simulink model "Sender"  (R2023a)
settings: Solver=FixedStepAuto  StartTime=0.0  StopTime=inf  RelTol=1e-3
undefined symbols (not defined in the file): DISTANCE, FINAL_1
libraries: androidaudiovideolib x4, simulink_extras x4, androidcommunicationlib x4, androiduilib x2, dspswit3 x2, androidsensorlib x2
settings Model: Creator=mohit  LastModifiedBy=mohit
settings OptimizationCC: EnhancedBackFolding=on  PassReuseOutputArgsAs=Individual arguments  ZeroExternalMemoryAtStartup=off  ZeroInternalMemoryAtStartup=off  MaxStackSize=64  OptimizeBlockOrder=speed  DifferentSizesBufferReuse=on  OptimizationCustomize=off  EfficientTunableParamExpr=on
settings DebuggingCC: ParameterTunabilityLossMsg=error
settings HardwareCC: ProdBitPerPointer=32  ProdBitPerSizeT=32  ProdBitPerPtrDiffT=32  ProdLargestAtomicInteger=Long  ProdLargestAtomicFloat=Double  ProdWordSize=32  ProdHWDeviceType=ARM Compatible->ARM Cortex  UseEmbeddedCoderFeatures=off  UseSimulinkCoderFeatures=off
settings SFSimCC: MATLABDynamicMemAlloc=off
settings RTWCC: Description=Embedded Coder  SystemTargetFile=ert.tlc  HardwareBoard=Android Device  TLCOptions="-aInlineSetEventsForThisBaseRateFcn=TLC_FALSE -aSuppressMultiTaskScheduler=TLC_FALSE  -aRateBasedStepFcn=0"  TemplateMakefile=ert_default_tmf  RTWVerbose=off  Toolchain=Android SDK/NDK Tools
settings CodeAppCC: ForceParamTrailComments=on  IgnoreCustomStorageClasses=off  OperatorAnnotations=on  SimulinkDataObjDesc=on  SFDataObjDesc=on  MangleLength=10  InsertBlockDesc=on
settings ERTTargetCC: SupportNonInlinedSFcns=on

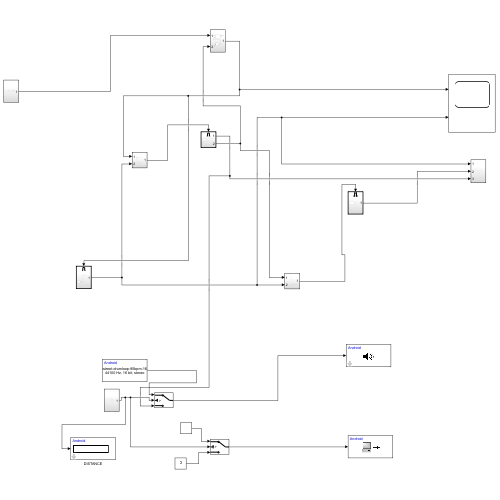
[thumbnail: Simulink's stored preview of the top-level diagram]
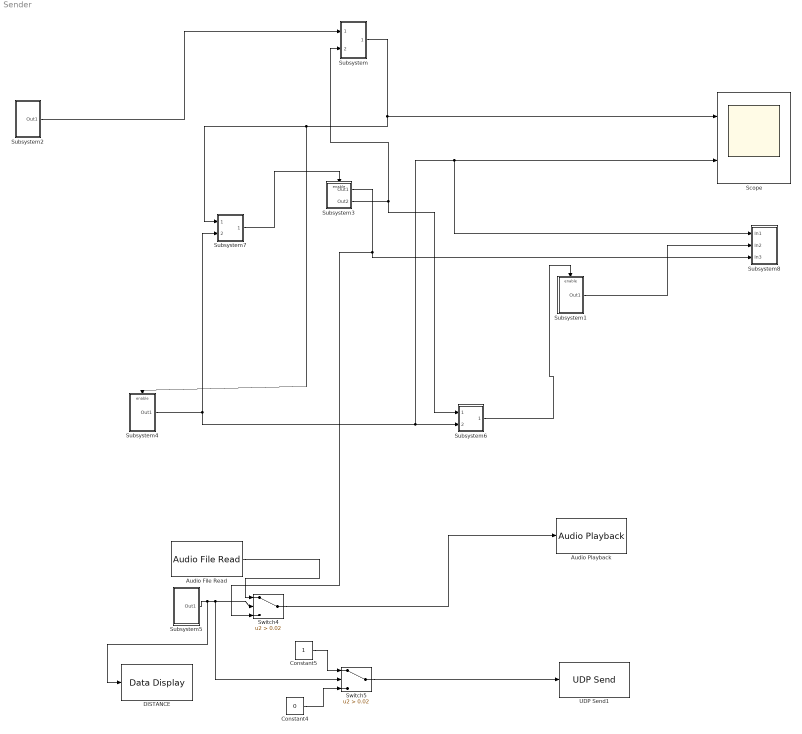
== system Sender ==
  Audio File Read : androidaudiovideolib/Audio File Read  FileName=C:\Users\mohit\OneDrive\Desktop\acad\ssrp\sunflower-street-drumloop-85bpm-163900.mp3  FrameSize=441
  Audio Playback : androidaudiovideolib/Audio Playback  SampleFreq=44100  AudioSamplingFreq=44100  SampleTime=0.1  DeviceStr=0  QueueDuration=0  BlockPlatform=Android
  Constant4 : Constant  Value=0  OutDataTypeStr=boolean
  Constant5 : Constant  OutDataTypeStr=boolean
  DISTANCE : androiduilib/Data Display  DataDisplayId=FINAL_1/DISTANCE  Format=Float  Precision=6  SimulateUsing=Code generation  blockPlatform=Android
  Scope : Scope  NumInputPorts=2
  Subsystem : Subsystem
  Subsystem1 : Subsystem
  Subsystem2 : Subsystem
  Subsystem3 : Subsystem
  Subsystem4 : Subsystem
  Subsystem5 : Subsystem
  Subsystem6 : Subsystem
  Subsystem7 : Subsystem
  Subsystem8 : Subsystem
  Switch4 : Switch  Criteria=u2 > Threshold  Threshold=0.02  OutDataTypeStr=int16  SaturateOnIntegerOverflow=off  InputSameDT=off
  Switch5 : Switch  Criteria=u2 > Threshold  Threshold=0.02  OutDataTypeStr=int16  SaturateOnIntegerOverflow=off  InputSameDT=off
  UDP Send1 : androidcommunicationlib/UDP Send  remoteURL='10.7.8.50'  remotePort=35000  localURL='0.0.0.0'  localPortSource=Automatically determine  localPort=-1  sampletime=-1  blockPlatform=Android  separateLengthPort=0
  wires:
  Subsystem2/1(Out1) -> Subsystem/1(In1)
  Subsystem4/1(Out1) -> Subsystem8/1(In1), Scope/2, Subsystem6/2(In2), Subsystem7/2(In2)
  Subsystem3/2(Out2) -> Subsystem/2(In2), Subsystem6/1(In1)
  Subsystem3/1(Out1) -> Subsystem8/3(In3), Switch4/3
  Subsystem/1(Out1) -> Subsystem7/1(In1), Subsystem4/Enable, Scope/1
  Audio File Read/1 -> Switch4/1
  Subsystem5/1(Out1) -> DISTANCE/1, Switch5/2, Switch4/2
  Constant4/1 -> Switch5/3
  Switch5/1 -> UDP Send1/1
  Constant5/1 -> Switch5/1
  Switch4/1 -> Audio Playback/1
  Subsystem6/1(Out1) -> Subsystem1/Enable
  Subsystem7/1(Out1) -> Subsystem3/Enable
  Subsystem1/1(Out1) -> Subsystem8/2(In2)

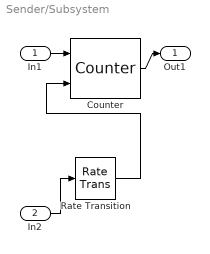
== system Sender/Subsystem ==
  In1 : Inport
  In2 : Inport  Port=2
  Counter : dspswit3/Counter  Direction=Up  CountEvent=Rising edge  CounterSize=16 bits  MaxCount=255  InitialCount=0  Output=Count  HitValue=1  ResetInput=on  SamplesPerFrame=1  Ts=1  CntDtype=double  HitDtype=Boolean
  Rate Transition : RateTransition
  Out1 : Outport
  wires:
  Rate Transition/1 -> Counter/2
  In1/1 -> Counter/1
  Counter/1 -> Out1/1
  In2/1 -> Rate Transition/1

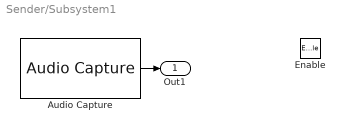
== system Sender/Subsystem1 ==
  Enable : EnablePort
  Audio Capture : androidaudiovideolib/Audio Capture  SampleFreq=44100  FrameSize=441  SampleTime=0.01  SimulateUsing=Code generation  DeviceStr=0  QueueDuration=0  BlockPlatform=Android  AudioSamplingFreq=44100
  Out1 : Outport
  wires:
  Audio Capture/1 -> Out1/1

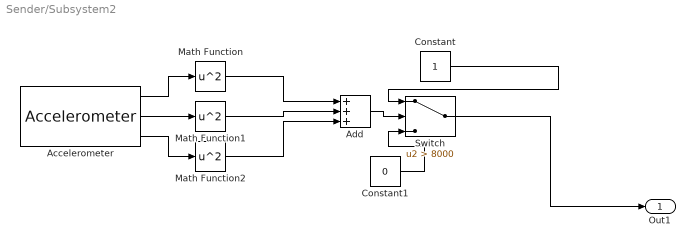
== system Sender/Subsystem2 ==
  Accelerometer : androidsensorlib/Accelerometer  OutputVector=off  SampleTime=0.02  BlockPlatform=Android
  Add : Sum  Inputs=+++
  Constant : Constant  OutDataTypeStr=int16
  Constant1 : Constant  Value=0  OutDataTypeStr=int16
  Math Function : Math  Operator=square
  Math Function1 : Math  Operator=square
  Math Function2 : Math  Operator=square
  Switch : Switch  Criteria=u2 > Threshold  Threshold=8000  SaturateOnIntegerOverflow=off  InputSameDT=off
  Out1 : Outport
  wires:
  Math Function/1 -> Add/1
  Constant1/1 -> Switch/3
  Math Function2/1 -> Add/3
  Math Function1/1 -> Add/2
  Constant/1 -> Switch/1
  Accelerometer/2 -> Math Function1/1
  Accelerometer/1 -> Math Function/1
  Accelerometer/3 -> Math Function2/1
  Add/1 -> Switch/2
  Switch/1 -> Out1/1

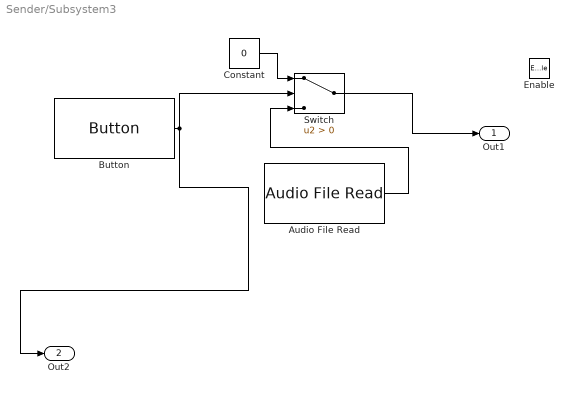
== system Sender/Subsystem3 ==
  Enable : EnablePort
  Audio File Read : androidaudiovideolib/Audio File Read  FileName=C:\Users\mohit\OneDrive\Desktop\acad\ssrp\file_example_WAV_1MG.wav  FrameSize=441
  Button : androiduilib/Button  ButtonState=Not pressed  ButtonId=FINAL_1/Subsystem3/Button  State=off  SampleTime=0.1  BlockPlatform=Android
  Constant : Constant  Value=0
  Switch : Switch  Criteria=u2 > Threshold  SaturateOnIntegerOverflow=off  InputSameDT=off
  Out1 : Outport
  Out2 : Outport  Port=2
  wires:
  Switch/1 -> Out1/1
  Button/1 -> Switch/2, Out2/1
  Audio File Read/1 -> Switch/3
  Constant/1 -> Switch/1

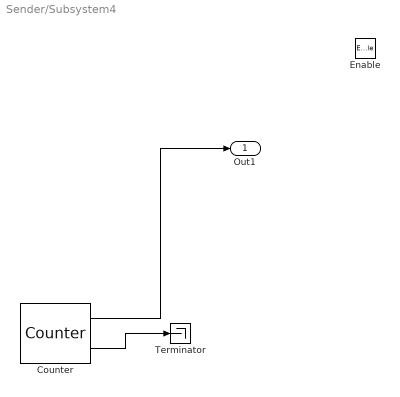
== system Sender/Subsystem4 ==
  Enable : EnablePort  StatesWhenEnabling=reset
  Counter : dspswit3/Counter  Direction=Up  CountEvent=Free running  CounterSize=16 bits  MaxCount=255  InitialCount=0  Output=Count and Hit  HitValue=5  ResetInput=off  SamplesPerFrame=1  Ts=1  CntDtype=double  HitDtype=Boolean
  Terminator : Terminator
  Out1 : Outport
  wires:
  Counter/1 -> Out1/1
  Counter/2 -> Terminator/1

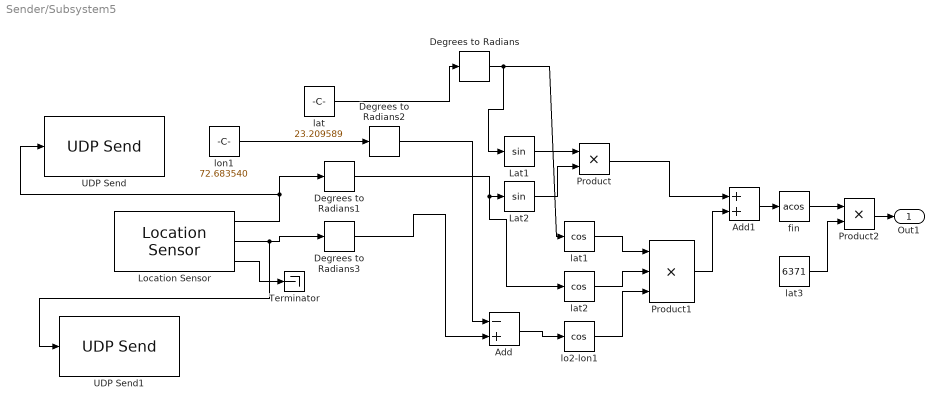
== system Sender/Subsystem5 ==
  Add : Sum  Inputs=-+
  Add1 : Sum
  Degrees to Radians{,1..3} (4 alike) : simulink_extras/Transformations/Degrees to Radians
  Lat1 : Trigonometry
  Lat2 : Trigonometry
  Location Sensor : androidsensorlib/Location Sensor  OutputVector=off  SampleTime=0.01  BlockPlatform=Android
  Product : Product
  Product1 : Product  Inputs=3
  Product2 : Product
  Terminator : Terminator
  UDP Send : androidcommunicationlib/UDP Send  remoteURL='10.7.8.50'  remotePort=30000  localURL='0.0.0.0'  localPortSource=Automatically determine  localPort=-1  sampletime=-1  blockPlatform=Android  separateLengthPort=0
  UDP Send1 : androidcommunicationlib/UDP Send  remoteURL='10.7.8.50'  remotePort=40000  localURL='0.0.0.0'  localPortSource=Automatically determine  localPort=-1  sampletime=-1  blockPlatform=Android  separateLengthPort=0
  fin : Trigonometry  Operator=acos
  lat : Constant  Value=23.209589
  lat1 : Trigonometry  Operator=cos
  lat2 : Trigonometry  Operator=cos
  lat3 : Constant  Value=6371
  lo2-lon1 : Trigonometry  Operator=cos
  lon1 : Constant  Value=72.683540
  Out1 : Outport
  wires:
  Product1/1 -> Add1/2
  Lat2/1 -> Product/2
  Degrees to Radians3/1 -> Add/2
  Degrees to Radians/1 -> Lat1/1, lat1/1
  Lat1/1 -> Product/1
  lo2-lon1/1 -> Product1/3
  lat3/1 -> Product2/2
  Product/1 -> Add1/1
  Degrees to Radians2/1 -> Add/1
  lat1/1 -> Product1/1
  lat2/1 -> Product1/2
  fin/1 -> Product2/1
  Location Sensor/1 -> UDP Send/1, Degrees to Radians1/1
  lat/1 -> Degrees to Radians/1
  lon1/1 -> Degrees to Radians2/1
  Add1/1 -> fin/1
  Location Sensor/2 -> UDP Send1/1, Degrees to Radians3/1
  Add/1 -> lo2-lon1/1
  Degrees to Radians1/1 -> lat2/1, Lat2/1
  Location Sensor/3 -> Terminator/1
  Product2/1 -> Out1/1

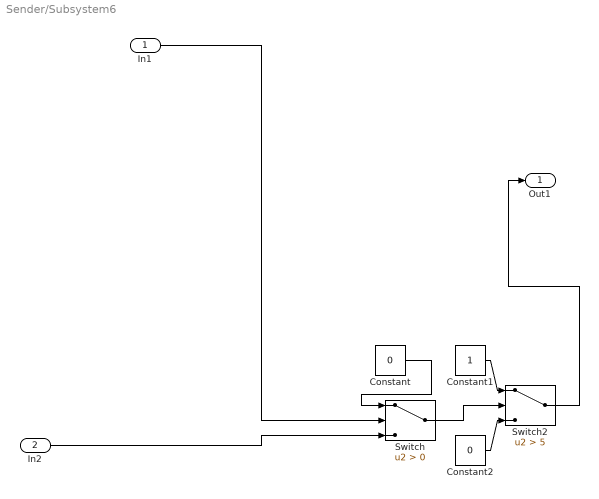
== system Sender/Subsystem6 ==
  In1 : Inport
  In2 : Inport  Port=2
  Constant : Constant  Value=0
  Constant1 : Constant
  Constant2 : Constant  Value=0
  Switch : Switch  Criteria=u2 > Threshold  SaturateOnIntegerOverflow=off  InputSameDT=off
  Switch2 : Switch  Criteria=u2 > Threshold  Threshold=5  OutDataTypeStr=int16  SaturateOnIntegerOverflow=off  InputSameDT=off
  Out1 : Outport
  wires:
  Constant2/1 -> Switch2/3
  Switch/1 -> Switch2/2
  Switch2/1 -> Out1/1
  Constant1/1 -> Switch2/1
  Constant/1 -> Switch/1
  In2/1 -> Switch/3
  In1/1 -> Switch/2

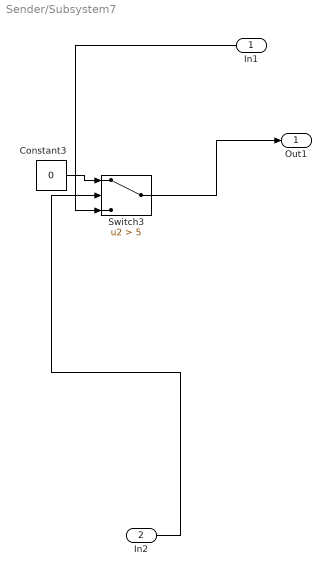
== system Sender/Subsystem7 ==
  In1 : Inport
  In2 : Inport  Port=2
  Constant3 : Constant  Value=0
  Switch3 : Switch  Criteria=u2 > Threshold  Threshold=5  OutDataTypeStr=int16  SaturateOnIntegerOverflow=off  InputSameDT=off
  Out1 : Outport
  wires:
  Constant3/1 -> Switch3/1
  In2/1 -> Switch3/2
  Switch3/1 -> Out1/1
  In1/1 -> Switch3/3

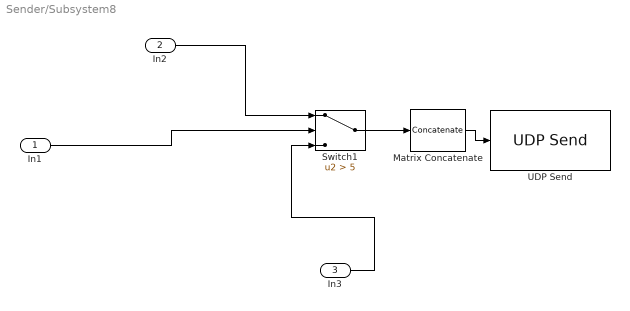
== system Sender/Subsystem8 ==
  In1 : Inport
  In2 : Inport  Port=2
  In3 : Inport  Port=3
  Matrix Concatenate : Concatenate  NumInputs=1  Mode=Multidimensional array  ConcatenateDimension=2
  Switch1 : Switch  Criteria=u2 > Threshold  Threshold=5  OutDataTypeStr=int16  SaturateOnIntegerOverflow=off  InputSameDT=off
  UDP Send : androidcommunicationlib/UDP Send  remoteURL='10.7.8.50'  remotePort=25000  localURL='0.0.0.0'  localPortSource=Automatically determine  localPort=-1  sampletime=-1  blockPlatform=Android  separateLengthPort=0
  wires:
  In3/1 -> Switch1/3
  Matrix Concatenate/1 -> UDP Send/1
  Switch1/1 -> Matrix Concatenate/1
  In1/1 -> Switch1/2
  In2/1 -> Switch1/1
